simulink model "ironer_line"  (R2020b)
settings: Solver=VariableStepAuto  StartTime=0.0  StopTime=20000  RelTol=1e-3
model workspace (MAT data in the model file):
  K1 = 43
  K_vv_o = 8.3
  K_vv_t = 1e-06
  M1 = 119
  M_vv_o = 1
  M_vv_t = 4.7
  R = 0.018
  Tank1_arb_offset = 707
  VV_o_arb_offset = 138
  V_roer_f = 9
  V_roer_t = 5
  c = 4180
undefined symbols (not defined in the file): D, EP_eff
libraries: simulink_extras x2, simulink x2, powerlib_meascontrol x1
settings Model: OrderedModelArguments=off  Creator=jonas  LastModifiedBy=Andreas
settings SolverCC: ZeroCrossAlgorithm=Adaptive
settings DebuggingCC: IgnoredZcDiagnostic=none

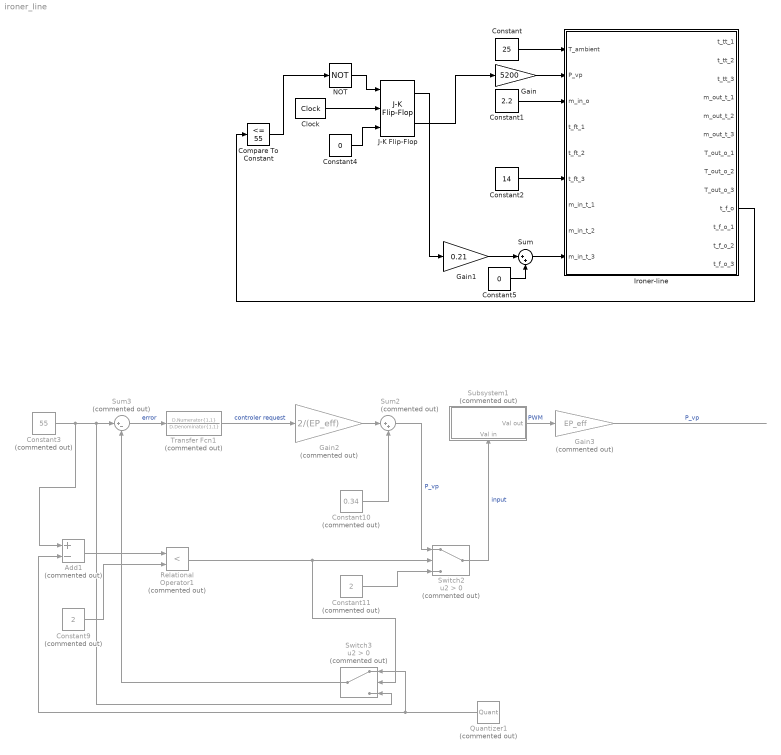
== system ironer_line ==
  Add1 : Sum  Commented=on  Inputs=+-
  Clock : simulink_extras/Flip Flops/Clock  period=1
  Compare To Constant : simulink/Logic and Bit Operations/Compare To Constant  relop=<=  const=55  OutDataTypeStr=boolean
  Constant : Constant  Value=25
  Constant1 : Constant  Value=2.2
  Constant10 : Constant  Commented=on  Value=0.34
  Constant11 : Constant  Commented=on  Value=2
  Constant2 : Constant  Value=14
  Constant3 : Constant  Commented=on  Value=55
  Constant4 : Constant  Value=0  OutDataTypeStr=boolean
  Constant5 : Constant  Value=0
  Constant9 : Constant  Commented=on  Value=2
  Gain : Gain  Gain=5200
  Gain1 : Gain  Gain=0.21
  Gain2 : Gain  Commented=on  Gain=2/(EP_eff)
  Gain3 : Gain  Commented=on  Gain=EP_eff
  Ironer-line : Subsystem
  J-K Flip-Flop : simulink_extras/Flip Flops/J-K Flip-Flop  initial_condition=0
  NOT : Logic  Operator=NOT  IconShape=distinctive  AllPortsSameDT=off  OutDataTypeStr=boolean
  Quantizer1 : Quantizer  Commented=on  QuantizationInterval=0.1  LinearizeAsGain=off
  Relational Operator1 : RelationalOperator  Commented=on  Operator=<  OutDataTypeStr=boolean  RndMeth=Simplest
  Subsystem1 : Subsystem  Commented=on
      settings: PortSchema="{\"entries\":[{\"content\":{\"sides\":[{\"content\":{\"connectorIds\":[]},\"type\":\"ConnectorPlacement.EquallySpacedRectSide\",\"uuid\":\"93d6448c-8be7-42d6-bbca-8ee67ab85f99\"},{\"content\":{\"connectorIds\":[\"Out1\"],\"side\":\"RIGHT\"},\"type\":\"ConnectorPlacement.EquallySpacedRectSide\",\"uuid\":\"d1f60a71-ea82-4b5d-adfc-1eb1997c4080\"},{\"content\":{\"connectorIds\":[],\"side\":\"TOP\"},\"type\":\"ConnectorPlacement.EquallySpacedRectSide\",\"uuid\":\"a17649c3-7f0c-44f8-8b19-4f62ca381b9d\"},{\"content\":{\"connectorIds\":[\"In1\"],\"side\":\"BOTTOM\"},\"type\":\"ConnectorPlacement.EquallySpacedRectSide\",\"uuid\":\"c02f8947-a6ab-4d8a-8dca-6adb48aadce7\"},{\"content\":{\"connectorIds\":[],\"side\":\"HIDDEN\"},\"type\":\"ConnectorPlacement.EquallySpacedRectSide\",\"uuid\":\"2a140053-ce1e-46d8-a035-c5351f3a00a7\"}]},\"type\":\"ConnectorPlacement.EquallySpacedConnector\",\"uuid\":\"b0b8ed38-8a01-4bf4-b4f7-dee60bb6f253\"}],\"packageUris\":[\"http://schema.mathworks.com/mf0/Connector/R2020b\"],\"version\":\"1.0\"}"
  Sum : Sum  Inputs=|++
  Sum2 : Sum  Commented=on  Inputs=|++
  Sum3 : Sum  Commented=on  Inputs=|+-
  Switch2 : Switch  Commented=on  Criteria=u2 > Threshold
  Switch3 : Switch  Commented=on  Criteria=u2 > Threshold
  Transfer Fcn1 : TransferFcn  Commented=on  Numerator=D.Numerator{1,1}  Denominator=D.Denominator{1,1}
  wires:
  Constant/1 -> Ironer-line/1(T_ambient)
  Constant1/1 -> Ironer-line/3(m_in_o)
  Constant2/1 -> Ironer-line/6(t_ft_3)
  Constant3/1 -> Add1/1, Switch3/3, Sum3/1
  ? -> Quantizer1/1
  Quantizer1/1 -> Switch3/1, Add1/2
  Add1/1 -> Relational Operator1/1
  Relational Operator1/1 -> Switch3/2, Switch2/2
  Constant9/1 -> Relational Operator1/2
  Sum2/1 -> Switch2/1  "P_vp"
  Switch3/1 -> Sum3/2
  Switch2/1 -> Subsystem1/1(Val in)  "input"
  Constant10/1 -> Sum2/2
  Transfer Fcn1/1 -> Gain2/1  "controler request"
  Constant11/1 -> Switch2/3
  Gain2/1 -> Sum2/1
  Sum3/1 -> Transfer Fcn1/1  "error"
  Gain3/1 -> ?  "P_vp"
  Subsystem1/1(Val out) -> Gain3/1  "PWM"
  Ironer-line/10(t_f_o) -> Compare To Constant/1
  Gain/1 -> Ironer-line/2(P_vp)
  Clock/1 -> J-K Flip-Flop/2
  Compare To Constant/1 -> NOT/1
  NOT/1 -> J-K Flip-Flop/1
  Constant4/1 -> J-K Flip-Flop/3
  J-K Flip-Flop/2 -> Gain/1
  J-K Flip-Flop/1 -> Gain1/1
  Gain1/1 -> Sum/1
  Constant5/1 -> Sum/2
  Sum/1 -> Ironer-line/9(m_in_t_3)

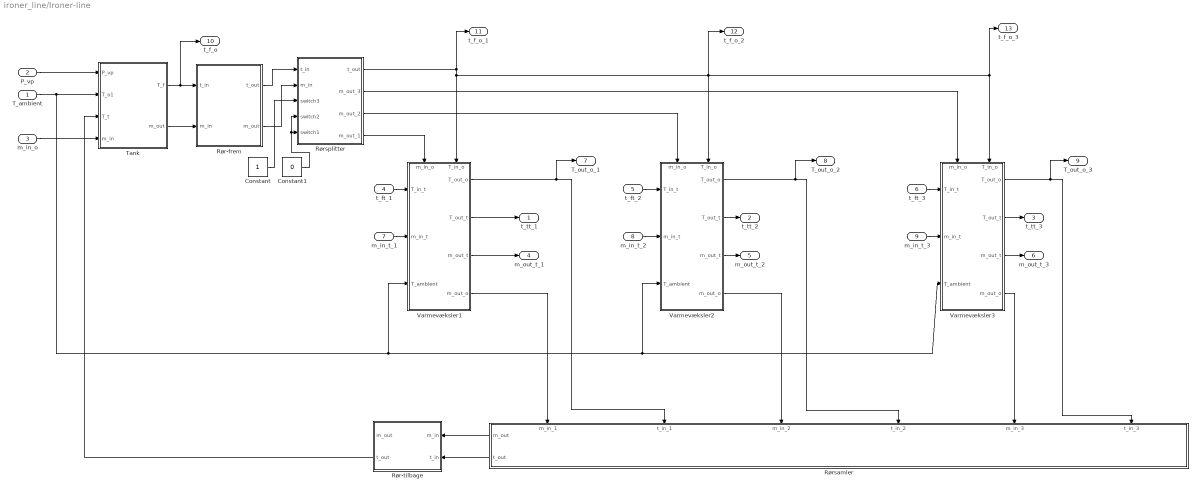
== system ironer_line/Ironer-line ==
  T_ambient : Inport
  P_vp : Inport  Port=2
  m_in_o : Inport  Port=3
  t_ft_1 : Inport  Port=4
  t_ft_2 : Inport  Port=5
  t_ft_3 : Inport  Port=6
  m_in_t_1 : Inport  Port=7
  m_in_t_2 : Inport  Port=8
  m_in_t_3 : Inport  Port=9
  Constant : Constant
  Constant1 : Constant  Value=0
  Rør-frem : Subsystem
  Rør-tilbage : Subsystem
  Rørsamler : Subsystem
      settings: PortSchema="{\"entries\":[{\"content\":{\"sides\":[{\"content\":{\"connectorIds\":[\"Out1\",\"Out2\"]},\"type\":\"ConnectorPlacement.EquallySpacedRectSide\",\"uuid\":\"ec17d99f-f8ae-471c-bafe-78515bbcabef\"},{\"content\":{\"connectorIds\":[],\"side\":\"RIGHT\"},\"type\":\"ConnectorPlacement.EquallySpacedRectSide\",\"uuid\":\"af5bd01a-b157-4ef9-a8b7-9f0f7cbff1fd\"},{\"content\":{\"connectorIds\":[\"In1\",\"In2\",\"In3\",\"In4\",\"In5\",\"In6\"],\"side\":\"TOP\"},\"type\":\"ConnectorPlacement.EquallySpacedRectSide\",\"uuid\":\"bf315a91-d0bc-423c-a297-1ceb99e4c009\"},{\"content\":{\"connectorIds\":[],\"side\":\"BOTTOM\"},\"type\":\"ConnectorPlacement.EquallySpacedRectSide\",\"uuid\":\"b7c90587-4528-4867-930a-87fdfb4fa087\"},{\"content\":{\"connectorIds\":[],\"side\":\"HIDDEN\"},\"type\":\"ConnectorPlacement.EquallySpacedRectSide\",\"uuid\":\"be1b6420-acd3-474c-9372-3b7276247edc\"}]},\"type\":\"ConnectorPlacement.EquallySpacedConnector\",\"uuid\":\"8133b3d7-d24a-478c-a0a4-73dbaad1198f\"}],\"packageUris\":[\"http://schema.mathworks.com/mf0/Connector/R2020b\"],\"version\":\"1.0\"}"
  Rørsplitter : Subsystem
  Tank : Subsystem
  Varmevæksler1 : Subsystem
      settings: PortSchema="{\"entries\":[{\"content\":{\"sides\":[{\"content\":{\"connectorIds\":[\"In1\",\"In2\",\"In3\"]},\"type\":\"ConnectorPlacement.EquallySpacedRectSide\",\"uuid\":\"883047e9-6272-4b1d-8029-8034b9d928d0\"},{\"content\":{\"connectorIds\":[\"Out1\",\"Out2\",\"Out3\",\"Out4\"],\"side\":\"RIGHT\"},\"type\":\"ConnectorPlacement.EquallySpacedRectSide\",\"uuid\":\"37325837-4c3d-4372-8e4e-b076780da32b\"},{\"content\":{\"connectorIds\":[\"In4\",\"In5\"],\"side\":\"TOP\"},\"type\":\"ConnectorPlacement.EquallySpacedRectSide\",\"uuid\":\"6f031f61-972f-41da-8329-b25e9d5b9b2e\"},{\"content\":{\"connectorIds\":[],\"side\":\"HIDDEN\"},\"type\":\"ConnectorPlacement.EquallySpacedRectSide\",\"uuid\":\"9f04c5b8-be80-4dbf-b80a-1de1f464f5f8\"}]},\"type\":\"ConnectorPlacement.EquallySpacedConnector\",\"uuid\":\"336a2d1e-6fb9-4225-890a-b0e1afffe7d3\"}],\"packageUris\":[\"http://schema.mathworks.com/mf0/Connector/R2020b\"],\"version\":\"1.0\"}"
  Varmevæksler2 : Subsystem
      settings: PortSchema="{\"entries\":[{\"content\":{\"sides\":[{\"content\":{\"connectorIds\":[\"In1\",\"In2\",\"In3\"]},\"type\":\"ConnectorPlacement.EquallySpacedRectSide\",\"uuid\":\"883047e9-6272-4b1d-8029-8034b9d928d0\"},{\"content\":{\"connectorIds\":[\"Out1\",\"Out2\",\"Out3\",\"Out4\"],\"side\":\"RIGHT\"},\"type\":\"ConnectorPlacement.EquallySpacedRectSide\",\"uuid\":\"37325837-4c3d-4372-8e4e-b076780da32b\"},{\"content\":{\"connectorIds\":[\"In4\",\"In5\"],\"side\":\"TOP\"},\"type\":\"ConnectorPlacement.EquallySpacedRectSide\",\"uuid\":\"6f031f61-972f-41da-8329-b25e9d5b9b2e\"},{\"content\":{\"connectorIds\":[],\"side\":\"HIDDEN\"},\"type\":\"ConnectorPlacement.EquallySpacedRectSide\",\"uuid\":\"9f04c5b8-be80-4dbf-b80a-1de1f464f5f8\"}]},\"type\":\"ConnectorPlacement.EquallySpacedConnector\",\"uuid\":\"336a2d1e-6fb9-4225-890a-b0e1afffe7d3\"}],\"packageUris\":[\"http://schema.mathworks.com/mf0/Connector/R2020b\"],\"version\":\"1.0\"}"
  Varmevæksler3 : Subsystem
      settings: PortSchema="{\"entries\":[{\"content\":{\"sides\":[{\"content\":{\"connectorIds\":[\"In1\",\"In2\",\"In3\"]},\"type\":\"ConnectorPlacement.EquallySpacedRectSide\",\"uuid\":\"883047e9-6272-4b1d-8029-8034b9d928d0\"},{\"content\":{\"connectorIds\":[\"Out1\",\"Out2\",\"Out3\",\"Out4\"],\"side\":\"RIGHT\"},\"type\":\"ConnectorPlacement.EquallySpacedRectSide\",\"uuid\":\"37325837-4c3d-4372-8e4e-b076780da32b\"},{\"content\":{\"connectorIds\":[\"In4\",\"In5\"],\"side\":\"TOP\"},\"type\":\"ConnectorPlacement.EquallySpacedRectSide\",\"uuid\":\"6f031f61-972f-41da-8329-b25e9d5b9b2e\"},{\"content\":{\"connectorIds\":[],\"side\":\"HIDDEN\"},\"type\":\"ConnectorPlacement.EquallySpacedRectSide\",\"uuid\":\"9f04c5b8-be80-4dbf-b80a-1de1f464f5f8\"}]},\"type\":\"ConnectorPlacement.EquallySpacedConnector\",\"uuid\":\"336a2d1e-6fb9-4225-890a-b0e1afffe7d3\"}],\"packageUris\":[\"http://schema.mathworks.com/mf0/Connector/R2020b\"],\"version\":\"1.0\"}"
  t_tt_1 : Outport
  t_tt_2 : Outport  Port=2
  t_tt_3 : Outport  Port=3
  m_out_t_1 : Outport  Port=4
  m_out_t_2 : Outport  Port=5
  m_out_t_3 : Outport  Port=6
  T_out_o_1 : Outport  Port=7
  T_out_o_2 : Outport  Port=8
  T_out_o_3 : Outport  Port=9
  t_f_o : Outport  Port=10
  t_f_o_1 : Outport  Port=11
  t_f_o_2 : Outport  Port=12
  t_f_o_3 : Outport  Port=13
  wires:
  P_vp/1 -> Tank/1(P_vp)
  Rørsplitter/1(t_out) -> Varmevæksler1/5(T_in_o), t_f_o_2/1, Varmevæksler2/5(T_in_o), Varmevæksler3/5(T_in_o), t_f_o_3/1, t_f_o_1/1
  t_ft_1/1 -> Varmevæksler1/1(T_in_t)
  t_ft_2/1 -> Varmevæksler2/1(T_in_t)
  t_ft_3/1 -> Varmevæksler3/1(T_in_t)
  Varmevæksler3/2(T_out_t) -> t_tt_3/1
  Varmevæksler2/2(T_out_t) -> t_tt_2/1
  Rørsplitter/4(m_out_1) -> Varmevæksler1/4(m_in_o)
  Rørsplitter/3(m_out_2) -> Varmevæksler2/4(m_in_o)
  Rørsplitter/2(m_out_3) -> Varmevæksler3/4(m_in_o)
  Varmevæksler1/2(T_out_t) -> t_tt_1/1
  T_ambient/1 -> Varmevæksler1/3(T_ambient), Varmevæksler3/3(T_ambient), Varmevæksler2/3(T_ambient), Tank/2(T_o1)
  m_in_t_1/1 -> Varmevæksler1/2(m_in_t)
  m_in_t_2/1 -> Varmevæksler2/2(m_in_t)
  m_in_t_3/1 -> Varmevæksler3/2(m_in_t)
  Varmevæksler1/3(m_out_t) -> m_out_t_1/1
  Varmevæksler2/3(m_out_t) -> m_out_t_2/1
  Varmevæksler3/3(m_out_t) -> m_out_t_3/1
  Varmevæksler1/4(m_out_o) -> Rørsamler/1(m_in_1)
  Varmevæksler1/1(T_out_o) -> T_out_o_1/1, Rørsamler/2(t_in_1)
  Varmevæksler2/4(m_out_o) -> Rørsamler/3(m_in_2)
  Varmevæksler3/4(m_out_o) -> Rørsamler/5(m_in_3)
  Varmevæksler3/1(T_out_o) -> T_out_o_3/1, Rørsamler/6(t_in_3)
  Rørsamler/1(m_out) -> Rør-tilbage/1(m_in)
  Rørsamler/2(t_out) -> Rør-tilbage/2(t_in)
  Rør-tilbage/2(t_out) -> Tank/3(T_t)
  Tank/2(m_out) -> Rør-frem/2(m_in)
  Rør-frem/2(m_out) -> Rørsplitter/2(m_in)
  Rør-frem/1(t_out) -> Rørsplitter/1(t_in)
  Tank/1(T_f) -> t_f_o/1, Rør-frem/1(t_in)
  m_in_o/1 -> Tank/4(m_in)
  Varmevæksler2/1(T_out_o) -> T_out_o_2/1, Rørsamler/4(t_in_2)
  Constant/1 -> Rørsplitter/3(switch3)
  Constant1/1 -> Rørsplitter/5(switch1), Rørsplitter/4(switch2)

== system ironer_line/Subsystem1 ==
  Val in : Inport
  Compare To Constant2 : simulink/Logic and Bit Operations/Compare To Constant  relop=<=  const=-1  OutDataTypeStr=boolean
  Subtract : Sum  Inputs=+-
  Triangle Generator : powerlib_meascontrol/Pulse & Signal Generators/Triangle Generator  Freq=0.2  Phase=0  Ts=0
  Zero-Order Hold : ZeroOrderHold  SampleTime=1/0.2
  Val out : Outport
  wires:
  Triangle Generator/1 -> Subtract/1
  Compare To Constant2/1 -> Val out/1
  Subtract/1 -> Compare To Constant2/1
  Val in/1 -> Zero-Order Hold/1
  Zero-Order Hold/1 -> Subtract/2

== system ironer_line/Ironer-line/Rør-frem ==
  t_in : Inport
  m_in : Inport  Port=2
  Constant : Constant  Value=V_roer_f
  Divide : Product  Inputs=*/
  Variable Time Delay : VariableTransportDelay  MaximumDelay=10
  t_out : Outport
  m_out : Outport  Port=2
  wires:
  t_in/1 -> Variable Time Delay/1
  Variable Time Delay/1 -> t_out/1
  m_in/1 -> m_out/1, Divide/2
  Constant/1 -> Divide/1
  Divide/1 -> Variable Time Delay/2

== system ironer_line/Ironer-line/Rør-tilbage ==
  m_in : Inport
  t_in : Inport  Port=2
  Constant : Constant  Value=V_roer_t
  Divide : Product  Inputs=*/
  Variable Time Delay : VariableTransportDelay  MaximumDelay=10
  m_out : Outport
  t_out : Outport  Port=2
  wires:
  t_in/1 -> Variable Time Delay/1
  Variable Time Delay/1 -> t_out/1
  Constant/1 -> Divide/1
  Divide/1 -> Variable Time Delay/2
  m_in/1 -> m_out/1, Divide/2

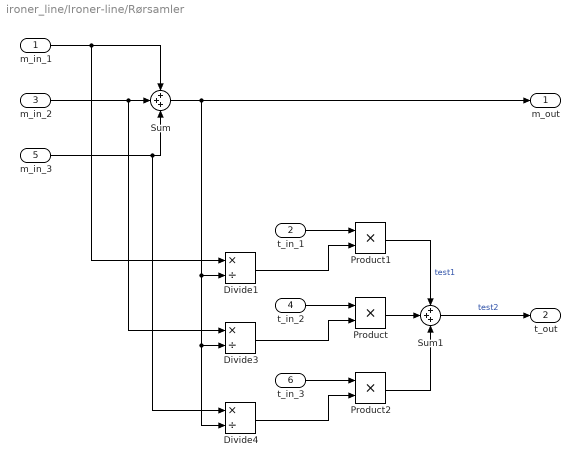
== system ironer_line/Ironer-line/Rørsamler ==
  m_in_1 : Inport
  t_in_1 : Inport  Port=2
  m_in_2 : Inport  Port=3
  t_in_2 : Inport  Port=4
  m_in_3 : Inport  Port=5
  t_in_3 : Inport  Port=6
  Divide1 : Product  Inputs=*/
  Divide3 : Product  Inputs=*/
  Divide4 : Product  Inputs=*/
  Product : Product
  Product1 : Product
  Product2 : Product
  Sum : Sum  Inputs=+++
  Sum1 : Sum  Inputs=+++
  m_out : Outport
  t_out : Outport  Port=2
  wires:
  m_in_1/1 -> Sum/1, Divide1/1
  m_in_2/1 -> Divide3/1, Sum/2
  m_in_3/1 -> Divide4/1, Sum/3
  t_in_1/1 -> Product1/1
  Product1/1 -> Sum1/1  "test1"
  Divide1/1 -> Product1/2
  Sum/1 -> m_out/1, Divide1/2, Divide4/2, Divide3/2
  t_in_2/1 -> Product/1
  Divide3/1 -> Product/2
  t_in_3/1 -> Product2/1
  Product2/1 -> Sum1/3
  Product/1 -> Sum1/2
  Divide4/1 -> Product2/2
  Sum1/1 -> t_out/1  "test2"

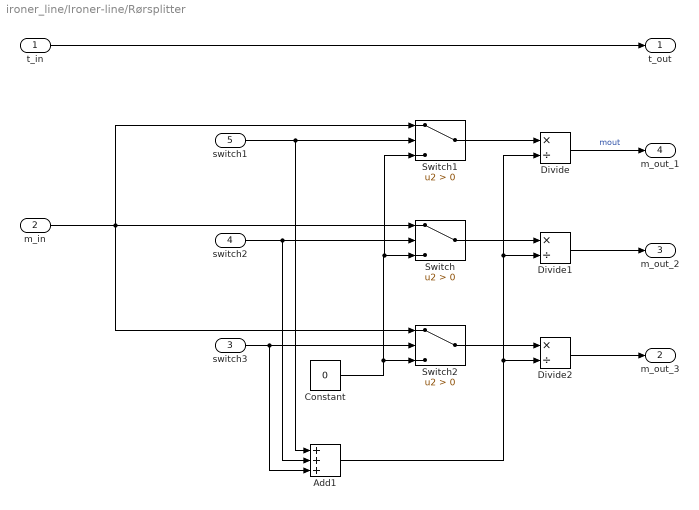
== system ironer_line/Ironer-line/Rørsplitter ==
  t_in : Inport
  m_in : Inport  Port=2
  switch3 : Inport  Port=3
  switch2 : Inport  Port=4
  switch1 : Inport  Port=5
  Add1 : Sum  Inputs=+++
  Constant : Constant  Value=0
  Divide : Product  Inputs=*/
  Divide1 : Product  Inputs=*/
  Divide2 : Product  Inputs=*/
  Switch : Switch  Criteria=u2 > Threshold
  Switch1 : Switch  Criteria=u2 > Threshold
  Switch2 : Switch  Criteria=u2 > Threshold
  t_out : Outport
  m_out_3 : Outport  Port=2
  m_out_2 : Outport  Port=3
  m_out_1 : Outport  Port=4
  wires:
  m_in/1 -> Switch1/1, Switch/1, Switch2/1
  t_in/1 -> t_out/1
  switch1/1 -> Add1/1, Switch1/2
  switch3/1 -> Add1/3, Switch2/2
  switch2/1 -> Add1/2, Switch/2
  Switch1/1 -> Divide/1
  Switch/1 -> Divide1/1
  Divide1/1 -> m_out_2/1
  Divide/1 -> m_out_1/1  "mout"
  Switch2/1 -> Divide2/1
  Divide2/1 -> m_out_3/1
  Constant/1 -> Switch1/3, Switch/3, Switch2/3
  Add1/1 -> Divide/2, Divide1/2, Divide2/2

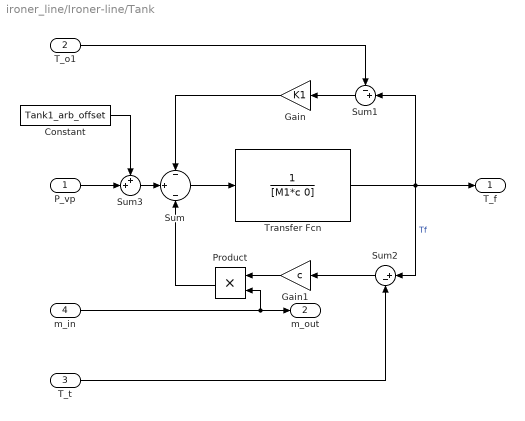
== system ironer_line/Ironer-line/Tank ==
  P_vp : Inport
  T_o1 : Inport  Port=2
  T_t : Inport  Port=3
  m_in : Inport  Port=4
  Constant : Constant  Value=Tank1_arb_offset
  Gain : Gain  Gain=K1
  Gain1 : Gain  Gain=c
  Product : Product
  Sum : Sum  Inputs=-|+|-
  Sum1 : Sum  Inputs=-+|
  Sum2 : Sum  Inputs=|+-
  Sum3 : Sum  Inputs=++|
  Transfer Fcn : TransferFcn  Denominator=[M1*c 0]
  T_f : Outport
  m_out : Outport  Port=2
  wires:
  T_o1/1 -> Sum1/1
  Sum1/1 -> Gain/1
  Sum/1 -> Transfer Fcn/1
  Transfer Fcn/1 -> T_f/1, Sum2/1, Sum1/2  "Tf"
  Gain/1 -> Sum/1
  T_t/1 -> Sum2/2
  Sum2/1 -> Gain1/1
  Gain1/1 -> Product/1
  Product/1 -> Sum/3
  m_in/1 -> m_out/1, Product/2
  Sum3/1 -> Sum/2
  P_vp/1 -> Sum3/2
  Constant/1 -> Sum3/1

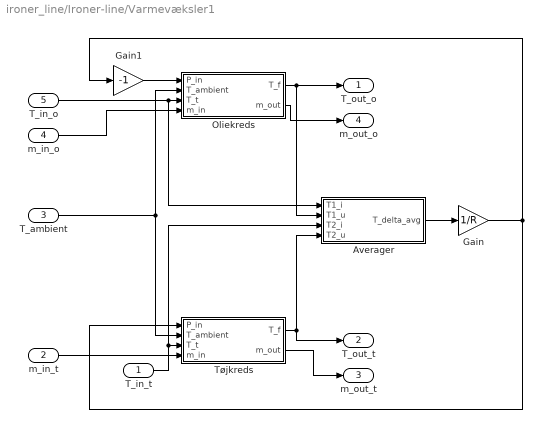
== system ironer_line/Ironer-line/Varmevæksler1 ==
  T_in_t : Inport
  m_in_t : Inport  Port=2
  T_ambient : Inport  Port=3
  m_in_o : Inport  Port=4
  T_in_o : Inport  Port=5
  Averager : Subsystem
  Gain : Gain  Gain=1/R
  Gain1 : Gain  Gain=-1
  Oliekreds : Subsystem
  Tøjkreds : Subsystem
  T_out_o : Outport
  T_out_t : Outport  Port=2
  m_out_t : Outport  Port=3
  m_out_o : Outport  Port=4
  wires:
  T_in_o/1 -> Averager/1(T1_i), Oliekreds/3(T_t)
  T_in_t/1 -> Averager/3(T2_i), Tøjkreds/3(T_t)
  Oliekreds/1(T_f) -> Averager/2(T1_u), T_out_o/1
  Tøjkreds/1(T_f) -> T_out_t/1, Averager/4(T2_u)
  Averager/1(T_delta_avg) -> Gain/1
  Gain1/1 -> Oliekreds/1(P_in)
  Gain/1 -> Tøjkreds/1(P_in), Gain1/1
  T_ambient/1 -> Tøjkreds/2(T_ambient), Oliekreds/2(T_ambient)
  m_in_o/1 -> Oliekreds/4(m_in)
  Oliekreds/2(m_out) -> m_out_o/1
  Tøjkreds/2(m_out) -> m_out_t/1
  m_in_t/1 -> Tøjkreds/4(m_in)

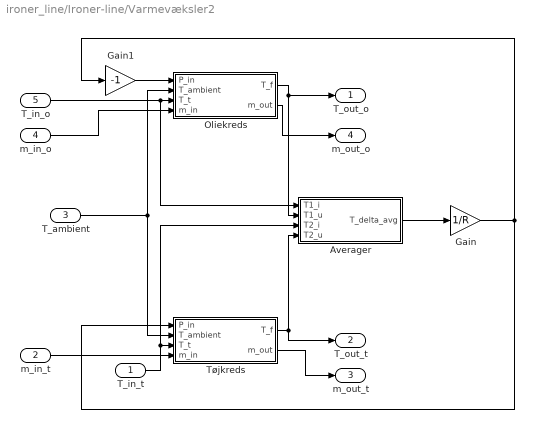
== system ironer_line/Ironer-line/Varmevæksler2 ==
  T_in_t : Inport
  m_in_t : Inport  Port=2
  T_ambient : Inport  Port=3
  m_in_o : Inport  Port=4
  T_in_o : Inport  Port=5
  Averager : Subsystem
  Gain : Gain  Gain=1/R
  Gain1 : Gain  Gain=-1
  Oliekreds : Subsystem
  Tøjkreds : Subsystem
  T_out_o : Outport
  T_out_t : Outport  Port=2
  m_out_t : Outport  Port=3
  m_out_o : Outport  Port=4
  wires:
  T_in_o/1 -> Averager/1(T1_i), Oliekreds/3(T_t)
  T_in_t/1 -> Averager/3(T2_i), Tøjkreds/3(T_t)
  Oliekreds/1(T_f) -> Averager/2(T1_u), T_out_o/1
  Tøjkreds/1(T_f) -> T_out_t/1, Averager/4(T2_u)
  Averager/1(T_delta_avg) -> Gain/1
  Gain1/1 -> Oliekreds/1(P_in)
  Gain/1 -> Tøjkreds/1(P_in), Gain1/1
  T_ambient/1 -> Tøjkreds/2(T_ambient), Oliekreds/2(T_ambient)
  m_in_o/1 -> Oliekreds/4(m_in)
  Oliekreds/2(m_out) -> m_out_o/1
  Tøjkreds/2(m_out) -> m_out_t/1
  m_in_t/1 -> Tøjkreds/4(m_in)

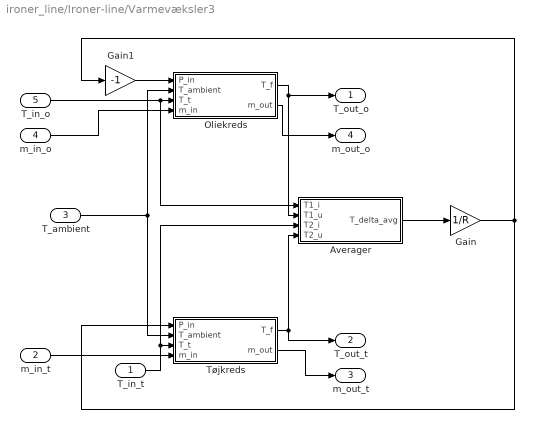
== system ironer_line/Ironer-line/Varmevæksler3 ==
  T_in_t : Inport
  m_in_t : Inport  Port=2
  T_ambient : Inport  Port=3
  m_in_o : Inport  Port=4
  T_in_o : Inport  Port=5
  Averager : Subsystem
  Gain : Gain  Gain=1/R
  Gain1 : Gain  Gain=-1
  Oliekreds : Subsystem
  Tøjkreds : Subsystem
  T_out_o : Outport
  T_out_t : Outport  Port=2
  m_out_t : Outport  Port=3
  m_out_o : Outport  Port=4
  wires:
  T_in_o/1 -> Averager/1(T1_i), Oliekreds/3(T_t)
  T_in_t/1 -> Averager/3(T2_i), Tøjkreds/3(T_t)
  Oliekreds/1(T_f) -> Averager/2(T1_u), T_out_o/1
  Tøjkreds/1(T_f) -> T_out_t/1, Averager/4(T2_u)
  Averager/1(T_delta_avg) -> Gain/1
  Gain1/1 -> Oliekreds/1(P_in)
  Gain/1 -> Tøjkreds/1(P_in), Gain1/1
  T_ambient/1 -> Tøjkreds/2(T_ambient), Oliekreds/2(T_ambient)
  m_in_o/1 -> Oliekreds/4(m_in)
  Oliekreds/2(m_out) -> m_out_o/1
  Tøjkreds/2(m_out) -> m_out_t/1
  m_in_t/1 -> Tøjkreds/4(m_in)

== system ironer_line/Ironer-line/Varmevæksler1/Averager ==
  T1_i : Inport
  T1_u : Inport  Port=2
  T2_i : Inport  Port=3
  T2_u : Inport  Port=4
  Gain : Gain  Gain=1/2
  Sum : Sum  Inputs=|++
  Sum1 : Sum  Inputs=++|
  Sum2 : Sum  Inputs=+-
  T_delta_avg : Outport
  wires:
  T1_u/1 -> Sum/1
  T1_i/1 -> Sum/2
  T2_i/1 -> Sum1/2
  T2_u/1 -> Sum1/1
  Sum1/1 -> Sum2/1
  Sum/1 -> Sum2/2
  Sum2/1 -> Gain/1
  Gain/1 -> T_delta_avg/1

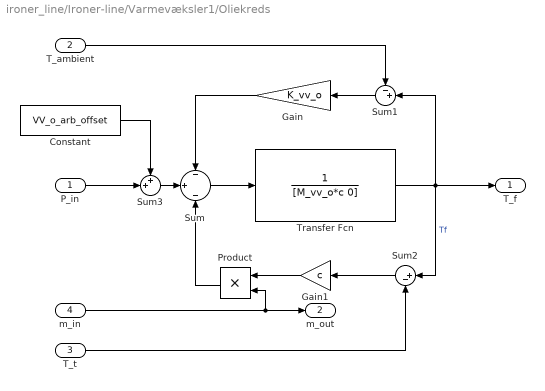
== system ironer_line/Ironer-line/Varmevæksler1/Oliekreds ==
  P_in : Inport
  T_ambient : Inport  Port=2
  T_t : Inport  Port=3
  m_in : Inport  Port=4
  Constant : Constant  Value=VV_o_arb_offset
  Gain : Gain  Gain=K_vv_o
  Gain1 : Gain  Gain=c
  Product : Product
  Sum : Sum  Inputs=-|+|-
  Sum1 : Sum  Inputs=-+|
  Sum2 : Sum  Inputs=|+-
  Sum3 : Sum  Inputs=++|
  Transfer Fcn : TransferFcn  Denominator=[M_vv_o*c 0]
  T_f : Outport
  m_out : Outport  Port=2
  wires:
  T_ambient/1 -> Sum1/1
  Sum1/1 -> Gain/1
  Sum/1 -> Transfer Fcn/1
  Transfer Fcn/1 -> T_f/1, Sum2/1, Sum1/2  "Tf"
  P_in/1 -> Sum3/2
  Gain/1 -> Sum/1
  T_t/1 -> Sum2/2
  Sum2/1 -> Gain1/1
  Gain1/1 -> Product/1
  Product/1 -> Sum/3
  m_in/1 -> m_out/1, Product/2
  Sum3/1 -> Sum/2
  Constant/1 -> Sum3/1

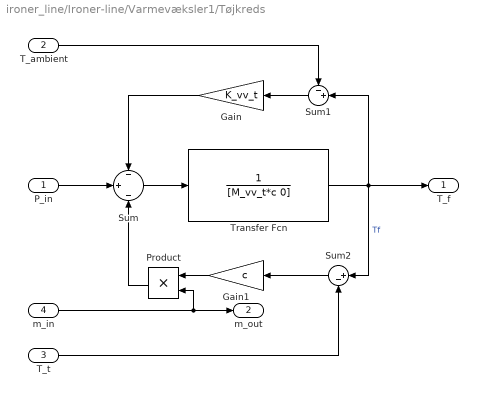
== system ironer_line/Ironer-line/Varmevæksler1/Tøjkreds ==
  P_in : Inport
  T_ambient : Inport  Port=2
  T_t : Inport  Port=3
  m_in : Inport  Port=4
  Gain : Gain  Gain=K_vv_t
  Gain1 : Gain  Gain=c
  Product : Product
  Sum : Sum  Inputs=-|+|-
  Sum1 : Sum  Inputs=-+|
  Sum2 : Sum  Inputs=|+-
  Transfer Fcn : TransferFcn  Denominator=[M_vv_t*c 0]
  T_f : Outport
  m_out : Outport  Port=2
  wires:
  T_ambient/1 -> Sum1/1
  Sum1/1 -> Gain/1
  Sum/1 -> Transfer Fcn/1
  Transfer Fcn/1 -> T_f/1, Sum2/1, Sum1/2  "Tf"
  P_in/1 -> Sum/2
  Gain/1 -> Sum/1
  T_t/1 -> Sum2/2
  Sum2/1 -> Gain1/1
  m_in/1 -> m_out/1, Product/2
  Gain1/1 -> Product/1
  Product/1 -> Sum/3

== system ironer_line/Ironer-line/Varmevæksler2/Averager ==
  T1_i : Inport
  T1_u : Inport  Port=2
  T2_i : Inport  Port=3
  T2_u : Inport  Port=4
  Gain : Gain  Gain=1/2
  Sum : Sum  Inputs=|++
  Sum1 : Sum  Inputs=++|
  Sum2 : Sum  Inputs=-+
  T_delta_avg : Outport
  wires:
  T1_u/1 -> Sum/1
  T1_i/1 -> Sum/2
  T2_i/1 -> Sum1/2
  T2_u/1 -> Sum1/1
  Sum1/1 -> Sum2/1
  Sum/1 -> Sum2/2
  Sum2/1 -> Gain/1
  Gain/1 -> T_delta_avg/1

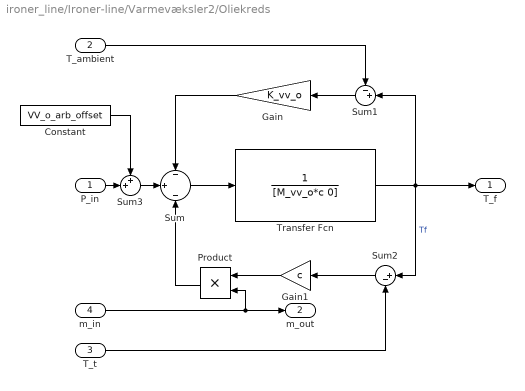
== system ironer_line/Ironer-line/Varmevæksler2/Oliekreds ==
  P_in : Inport
  T_ambient : Inport  Port=2
  T_t : Inport  Port=3
  m_in : Inport  Port=4
  Constant : Constant  Value=VV_o_arb_offset
  Gain : Gain  Gain=K_vv_o
  Gain1 : Gain  Gain=c
  Product : Product
  Sum : Sum  Inputs=-|+|-
  Sum1 : Sum  Inputs=-+|
  Sum2 : Sum  Inputs=|+-
  Sum3 : Sum  Inputs=++|
  Transfer Fcn : TransferFcn  Denominator=[M_vv_o*c 0]
  T_f : Outport
  m_out : Outport  Port=2
  wires:
  T_ambient/1 -> Sum1/1
  Sum1/1 -> Gain/1
  Sum/1 -> Transfer Fcn/1
  Transfer Fcn/1 -> T_f/1, Sum2/1, Sum1/2  "Tf"
  P_in/1 -> Sum3/2
  Gain/1 -> Sum/1
  T_t/1 -> Sum2/2
  Sum2/1 -> Gain1/1
  Gain1/1 -> Product/1
  Product/1 -> Sum/3
  m_in/1 -> m_out/1, Product/2
  Constant/1 -> Sum3/1
  Sum3/1 -> Sum/2

== system ironer_line/Ironer-line/Varmevæksler2/Tøjkreds ==
  P_in : Inport
  T_ambient : Inport  Port=2
  T_t : Inport  Port=3
  m_in : Inport  Port=4
  Gain : Gain  Gain=K_vv_t
  Gain1 : Gain  Gain=c
  Product : Product
  Sum : Sum  Inputs=-|+|-
  Sum1 : Sum  Inputs=-+|
  Sum2 : Sum  Inputs=|+-
  Transfer Fcn : TransferFcn  Denominator=[M_vv_t*c 0]
  T_f : Outport
  m_out : Outport  Port=2
  wires:
  T_ambient/1 -> Sum1/1
  Sum1/1 -> Gain/1
  Sum/1 -> Transfer Fcn/1
  Transfer Fcn/1 -> T_f/1, Sum2/1, Sum1/2  "Tf"
  P_in/1 -> Sum/2
  Gain/1 -> Sum/1
  T_t/1 -> Sum2/2
  Sum2/1 -> Gain1/1
  m_in/1 -> m_out/1, Product/2
  Gain1/1 -> Product/1
  Product/1 -> Sum/3

== system ironer_line/Ironer-line/Varmevæksler3/Averager ==
  T1_i : Inport
  T1_u : Inport  Port=2
  T2_i : Inport  Port=3
  T2_u : Inport  Port=4
  Gain : Gain  Gain=1/2
  Sum : Sum  Inputs=|++
  Sum1 : Sum  Inputs=++|
  Sum2 : Sum  Inputs=-+
  T_delta_avg : Outport
  wires:
  T1_u/1 -> Sum/1
  T1_i/1 -> Sum/2
  T2_i/1 -> Sum1/2
  T2_u/1 -> Sum1/1
  Sum1/1 -> Sum2/1
  Sum/1 -> Sum2/2
  Sum2/1 -> Gain/1
  Gain/1 -> T_delta_avg/1

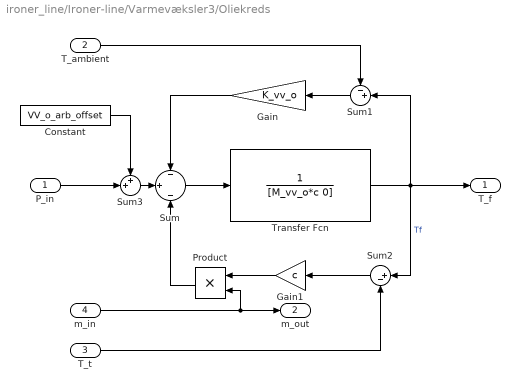
== system ironer_line/Ironer-line/Varmevæksler3/Oliekreds ==
  P_in : Inport
  T_ambient : Inport  Port=2
  T_t : Inport  Port=3
  m_in : Inport  Port=4
  Constant : Constant  Value=VV_o_arb_offset
  Gain : Gain  Gain=K_vv_o
  Gain1 : Gain  Gain=c
  Product : Product
  Sum : Sum  Inputs=-|+|-
  Sum1 : Sum  Inputs=-+|
  Sum2 : Sum  Inputs=|+-
  Sum3 : Sum  Inputs=++|
  Transfer Fcn : TransferFcn  Denominator=[M_vv_o*c 0]
  T_f : Outport
  m_out : Outport  Port=2
  wires:
  T_ambient/1 -> Sum1/1
  Sum1/1 -> Gain/1
  Sum/1 -> Transfer Fcn/1
  Transfer Fcn/1 -> T_f/1, Sum2/1, Sum1/2  "Tf"
  P_in/1 -> Sum3/2
  Gain/1 -> Sum/1
  T_t/1 -> Sum2/2
  Sum2/1 -> Gain1/1
  Gain1/1 -> Product/1
  Product/1 -> Sum/3
  m_in/1 -> m_out/1, Product/2
  Constant/1 -> Sum3/1
  Sum3/1 -> Sum/2

== system ironer_line/Ironer-line/Varmevæksler3/Tøjkreds ==
  P_in : Inport
  T_ambient : Inport  Port=2
  T_t : Inport  Port=3
  m_in : Inport  Port=4
  Gain : Gain  Gain=K_vv_t
  Gain1 : Gain  Gain=c
  Product : Product
  Sum : Sum  Inputs=-|+|-
  Sum1 : Sum  Inputs=-+|
  Sum2 : Sum  Inputs=|+-
  Transfer Fcn : TransferFcn  Denominator=[M_vv_t*c 0]
  T_f : Outport
  m_out : Outport  Port=2
  wires:
  T_ambient/1 -> Sum1/1
  Sum1/1 -> Gain/1
  Sum/1 -> Transfer Fcn/1
  Transfer Fcn/1 -> T_f/1, Sum2/1, Sum1/2  "Tf"
  P_in/1 -> Sum/2
  Gain/1 -> Sum/1
  T_t/1 -> Sum2/2
  Sum2/1 -> Gain1/1
  m_in/1 -> m_out/1, Product/2
  Gain1/1 -> Product/1
  Product/1 -> Sum/3
